simulink model "PID_Simulink_con_ventilador_R2021b"  (R2021b)
settings: Solver=ode3  StartTime=0.0  StopTime=600  RelTol=1e-3  EnableMultiTasking=on
undefined symbols (not defined in the file): T
libraries: arduinolib x4
settings Model: FPTRunName=Active  ExtModeTrigDuration=2  Creator=The MathWorks, Inc.  LastModifiedBy=JOSEJUAN
settings SolverCC: AlgebraicLoopSolver=TrustRegion
settings DataIOCC: LimitDataPoints=on  SaveFormat=Array  ReturnWorkspaceOutputs=off
settings OptimizationCC: ExpressionDepthLimit=2147483647  LifeSpan=Inf  MaxStackSize=64
settings DebuggingCC: UnderspecifiedInitializationDetection=Classic  MergeDetectMultiDrivingBlocksExec=none  FcnCallInpInsideContextMsg=warning  AllowSymbolicDim=off  StateNameClashWarn=warning  SFUnexpectedBacktrackingDiag=warning  SFNoUnconditionalDefaultTransitionDiag=warning  SFExecutionAtInitializationDiag=none  SFMachineParentedDataDiag=warning  ArithmeticOperatorsInVariantConditions=warning
settings HardwareCC: ProdBitPerInt=16  ProdBitPerPointer=16  ProdBitPerSizeT=16  ProdBitPerPtrDiffT=16  ProdLargestAtomicFloat=None  ProdWordSize=8  ProdHWDeviceType=Atmel->AVR
settings ModelReferenceCC: PropagateSignalLabelsOutOfModel=off
settings SFSimCC: SimUseLocalCustomCode=off  MATLABDynamicMemAlloc=off
settings RTWCC: Description=Embedded Coder  SystemTargetFile=ert.tlc  HardwareBoard=Arduino Uno  TemplateMakefile=ert_default_tmf  GenerateReport=on  RTWVerbose=off  RTWUseLocalCustomCode=off  Toolchain=Arduino AVR  BuildConfiguration=Faster Runs  LaunchReport=on
settings CodeAppCC: ForceParamTrailComments=on  OperatorAnnotations=on  StateflowObjectComments=on  MATLABSourceComments=on
settings ERTTargetCC: MultiwordLength=2048  ERTCustomFileBanners=off  SupportContinuousTime=on  SupportNonInlinedSFcns=on  RemoveResetFunc=off  SupportVariableSizeSignals=on  ModelStepFunctionPrototypeControlCompliant=off  ExtModeStaticAllocSize=250
settings ConfigComp: CovMetricSettings=dw  CovSaveCumulativeToWorkspaceVar=on  CovSaveSingleToWorkspaceVar=on  CovExternalEMLEnable=off  CovSFcnEnable=off

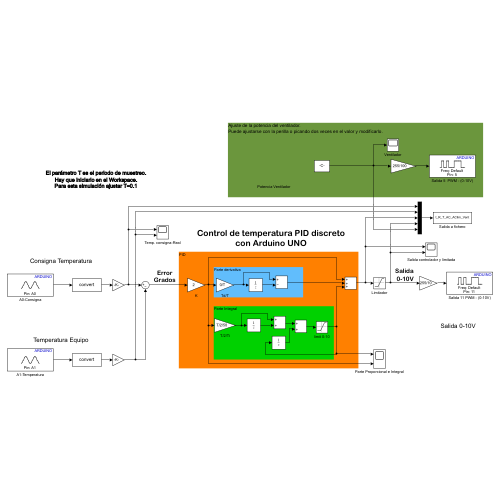
[thumbnail: Simulink's stored preview of the top-level diagram]
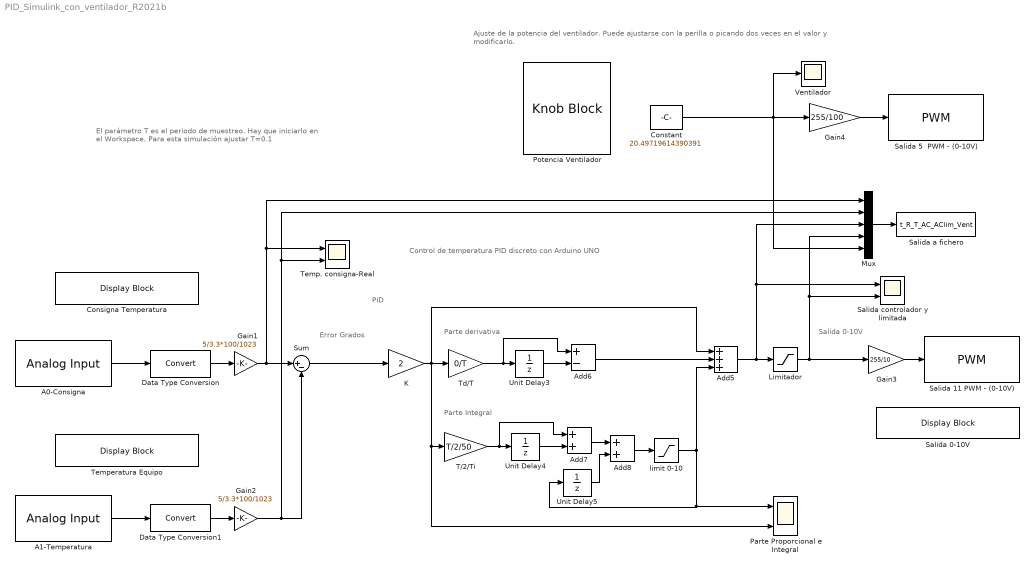
== system PID_Simulink_con_ventilador_R2021b ==
  note: El parámetro T es el periodo de muestreo.
      | Hay que iniciarlo en el Workspace.
      | Para esta simulación ajustar T=0.1
  note: Control de temperatura PID discreto
      | con Arduino UNO
  note: PID
  note: Error
      | Grados
  note: Salida
      | 0-10V
  note: Parte derivativa
  note: Parte Integral
  note: Ajuste de la potencia del ventilador.
      | Puede ajustarse con la perilla o picando dos veces en el valor y modificarlo.
  A0-Consigna : arduinolib/Analog Input  pinNumber=0  ReadResultsOnly=off  ConversionTriggerSource=Software  ExternalTriggerType=uint32( 0 )  OutputDataType=uint16  EnableConversionCompleteNotify=off  EnableOuputStatus=off  SampleTime=T  blockPlatform=arduino
  A1-Temperatura : arduinolib/Analog Input  pinNumber=1  ReadResultsOnly=off  ConversionTriggerSource=Software  ExternalTriggerType=uint32( 0 )  OutputDataType=uint16  EnableConversionCompleteNotify=off  EnableOuputStatus=off  SampleTime=T  blockPlatform=arduino
  Add5 : Sum  Inputs=+++
  Add6 : Sum  Inputs=+-
  Add7 : Sum
  Add8 : Sum
  Consigna Temperatura : DisplayBlock  LabelPosition=Hide  Format=bank  Transparency=1
  Constant : Constant  Value=20.49719614390391  SampleTime=T
  Data Type Conversion : DataTypeConversion
  Data Type Conversion1 : DataTypeConversion
  Gain1 : Gain  Gain=5/3.3*100/1023
  Gain2 : Gain  Gain=5/3.3*100/1023
  Gain3 : Gain  Gain=255/10
  Gain4 : Gain  Gain=255/100
  K : Gain  Gain=2
  Limitador : Saturate  UpperLimit=10  LowerLimit=0
  Mux : Mux  Inputs=5
  Parte Proporcional e Integral : Scope  NumInputPorts=2
  Potencia Ventilador : KnobBlock
  Salida 0-10V : DisplayBlock  LabelPosition=Hide  Format=Integer  Transparency=1
  Salida 11 PWM - (0-10V) : arduinolib/PWM  pinNumber=11  frequencyType=Default  desiredFrequency=490.2  achievableFrequency=490.2
  Salida 5  PWM - (0-10V) : arduinolib/PWM  pinNumber=5  frequencyType=Default  desiredFrequency=490.2  achievableFrequency=490.2
  Salida a fichero : ToFile  Filename=t_R_T_AC_AClim_Vent  MatrixName=t_R_T_AC_AClim  SaveFormat=Timeseries
  Salida controlador y limitada : Scope  NumInputPorts=2
  Sum : Sum  Inputs=|+-
  T/2/Ti : Gain  Gain=T/2/50
  Td/T : Gain  Gain=0/T
  Temp. consigna-Real : Scope  NumInputPorts=2
  Temperatura Equipo : DisplayBlock  LabelPosition=Hide  Format=bank  Transparency=1
  Unit Delay3 : UnitDelay  SampleTime=T  HasFrameUpgradeWarning=on
  Unit Delay4 : UnitDelay  SampleTime=T  HasFrameUpgradeWarning=on
  Unit Delay5 : UnitDelay  SampleTime=T  HasFrameUpgradeWarning=on
  Ventilador : Scope
  limit 0-10 : Saturate  UpperLimit=10*1.0  LowerLimit=0
  wires:
  A0-Consigna/1 -> Data Type Conversion/1
  A1-Temperatura/1 -> Data Type Conversion1/1
  Gain3/1 -> Salida 11 PWM - (0-10V)/1
  Sum/1 -> K/1
  Data Type Conversion1/1 -> Gain2/1
  Data Type Conversion/1 -> Gain1/1
  Gain1/1 -> Sum/1, Temp. consigna-Real/1, Mux/1
  Gain2/1 -> Temp. consigna-Real/2, Mux/2, Sum/2
  Add6/1 -> Add5/2
  Add8/1 -> limit 0-10/1
  limit 0-10/1 -> Add5/3, Unit Delay5/1, Parte Proporcional e Integral/1
  Unit Delay5/1 -> Add8/2
  K/1 -> T/2/Ti/1, Parte Proporcional e Integral/2, Add5/1, Td/T/1
  T/2/Ti/1 -> Add7/1, Unit Delay4/1
  Add7/1 -> Add8/1
  Unit Delay3/1 -> Add6/2
  Td/T/1 -> Unit Delay3/1, Add6/1
  Unit Delay4/1 -> Add7/2
  Add5/1 -> Limitador/1, Salida controlador y limitada/1, Mux/3
  Mux/1 -> Salida a fichero/1
  Limitador/1 -> Gain3/1, Salida controlador y limitada/2, Mux/4
  Gain4/1 -> Salida 5  PWM - (0-10V)/1
  Constant/1 -> Ventilador/1, Gain4/1, Mux/5
